simulink model "CF010A_GmTqArbn"  (R2013b)
settings: Solver=FixedStepDiscrete  SolverMode=SingleTasking  StartTime=0.0  StopTime=1  FixedStep=0.002  RelTol=1e-3
values from neighbouring files (symbols this model uses):
  ARCHGLBPRM_2MILLISEC_SEC_F32 = DataDict.Constant    [CF010A_GmTqArbn_DataDict.m]
  ESCTQCMDOVRLLIM_HWNWTMTR_F32 = DataDict.Constant    [CF010A_GmTqArbn_DataDict.m]
  FINALSLEWLWRLIM_HWNWTMTRPERSEC_F32 = DataDict.Constant    [CF010A_GmTqArbn_DataDict.m]
  GmTqArbnApaAssiScaEna = DataDict.Calibration    [CF010A_GmTqArbn_DataDict.m]
  GmTqArbnApaDampgScaEna = DataDict.Calibration    [CF010A_GmTqArbn_DataDict.m]
  GmTqArbnApaEnaRate = DataDict.Calibration    [CF010A_GmTqArbn_DataDict.m]
  GmTqArbnApaRtnScaEna = DataDict.Calibration    [CF010A_GmTqArbn_DataDict.m]
  GmTqArbnEscMaxTq = DataDict.Calibration    [CF010A_GmTqArbn_DataDict.m]
  GmTqArbnLkaOutpOvrlUpprLim = DataDict.Calibration    [CF010A_GmTqArbn_DataDict.m]
  GmTqArbnLkaSlewEna = DataDict.Calibration    [CF010A_GmTqArbn_DataDict.m]
  HWTQCMDOVRLLIM_HWNWTMTR_F32 = DataDict.Constant    [CF010A_GmTqArbn_DataDict.m]
  LKACMDHILIM_HWNWTMTR_F32 = DataDict.Constant    [CF010A_GmTqArbn_DataDict.m]
  LKAOUTPOVRLLIM_MOTNWTMTR_F32 = DataDict.Constant    [CF010A_GmTqArbn_DataDict.m]
  LKATQCMDOVRLLIM_HWNWTMTR_F32 = DataDict.Constant    [CF010A_GmTqArbn_DataDict.m]
  MOTTQCMDOVRLLIM_MOTNWTMTR_F32 = DataDict.Constant    [CF010A_GmTqArbn_DataDict.m]
  OUTPCMDHILIM_ULS_F32 = DataDict.Constant    [CF010A_GmTqArbn_DataDict.m]
  OUTPCMDLOWRLIM_ULS_F32 = DataDict.Constant    [CF010A_GmTqArbn_DataDict.m]
  POSNSERVOSMOOTHMINLWRLIM_ULSPERSEC_F32 = DataDict.Constant    [CF010A_GmTqArbn_DataDict.m]
  VELDPTTQOVRLMTRCOFFS_HWNWTMTRPERSEC_F32 = DataDict.Constant    [CF010A_GmTqArbn_DataDict.m]
  VELDPTTQOVRLMTRCTQPERVEHSPD_HWNWTMTRPERSECPERKPH_F32 = DataDict.Constant    [CF010A_GmTqArbn_DataDict.m]
undefined symbols (not defined in the file or in its folder): GmTqArbnEscSt1, GmTqArbnLkaSt1
libraries: NxtrLim x12, simulink x10, NexteerUtilities x8, FixdToFloat x4, NxtrAbslt x3, Fil x2, FloatToFixd x2, BilnrIntrpnMplX x1, NxtrSign x1
(part 3 of 5)

== system CF010A_GmTqArbn/call_GmTqArbnInit1/Subsystem5 ==

== system CF010A_GmTqArbn/call_GmTqArbnPer1/Subsystem5 ==

== system CF010A_GmTqArbn/GmTqArbn/GmTqArbnInit1/CopyRight2 ==

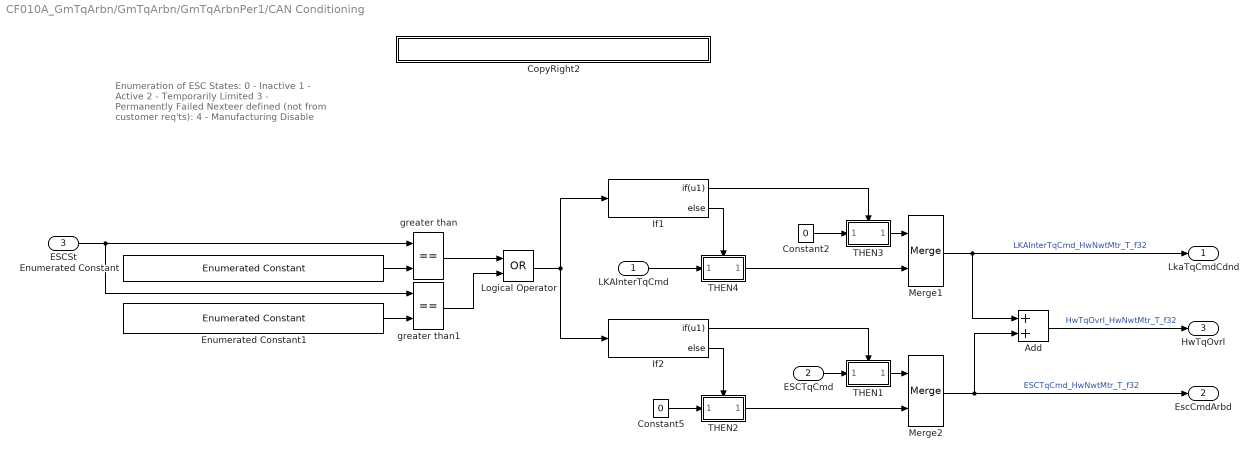
== system CF010A_GmTqArbn/GmTqArbn/GmTqArbnPer1/CAN Conditioning ==
  note: Enumeration of ESC States:
      |     0 - Inactive
      |     1 - Active
      |     2 - Temporarily Limited
      |     3 - Permanently Failed
      |
      | Nexteer defined (not from customer req'ts):
      |     4 - Manufacturing Disable
  LKAInterTqCmd : Inport
  ESCTqCmd : Inport  Port=2
  ESCSt : Inport  Port=3
  Add : Sum
  Constant2 : Constant  Value=0  OutDataTypeStr=single
  Constant5 : Constant  Value=0  OutDataTypeStr=single
  CopyRight2 : Subsystem  Description=|  mask(Copyright Information){none=on}
      | Copyright info block.                                               
      |                                                                     
      | Place copyright information at the top of every subsystem in design.
      mask prompts: none "No parameters"
      mask help: Place copyright information at the top of every subsystem in design.
      mask Display:
      | NxtrConf = 'Nexteer Confidential';
      | 
      | sys = bdroot; %handle for the current model ("system")
      | first = get_param(sys,'Created');
      | first = first(end-3:end);  %year is last four digits
      | 
      | last = get_param(sys,'LastModifiedDate');
      | if isempty(last)
      |     last = datestr(now,'yyyy');
      | else
      |     last = last(end-3:end);
      | end
      | 
      | if strcmp(first,last)
      |     fprintf('%s -- Copyright %s Nexteer',NxtrConf,first)
      | else
      |     fprintf('%s -- %s%s- %s Nexteer',NxtrConf,char(169),first,last)
      | end
  Enumerated Constant : simulink/Sources/Enumerated Constant  OutDataTypeStr=Enum: GmTqArbnEscSt1  Value=GmTqArbnEscSt1.GMTQARBNESCST_ACTV  SampleTime=inf
  Enumerated Constant1 : simulink/Sources/Enumerated Constant  OutDataTypeStr=Enum: GmTqArbnEscSt1  Value=GmTqArbnEscSt1.GMTQARBNESCST_TMPLIMD  SampleTime=inf
  If1 : If  IfExpression=u1
  If2 : If  IfExpression=u1
  Logical Operator : Logic  Operator=OR  AllPortsSameDT=off  OutDataTypeStr=boolean
  Merge1 : Merge
  Merge2 : Merge
  THEN1 : Subsystem  RequirementInfo={} %GIDa_df789066_5626_4b2f_a61b_8784029d3cc8  TreatAsAtomicUnit=on  mask(pass thru, version Nov 30, 2012){nIn=1}
      mask prompts: nIn "Number of input signals"
      mask help:
      | This block passes its input straight through without modification.
      |
      | Enter the number of signals to pass through (integer 1 to 5).
      mask Callback nIn:
      | thisBlock = gcb;
      | a = get_param(thisBlock,'MaskValues');
      | b = cell2mat(a);
      | c = str2num(b);
      | 
      | if c<1 c=1; end
      | if c>5 c=5; end
      | 
      | for idx=1:c
      |     sIdx = num2str(idx);
      |     oldblock = [thisBlock '/In' sIdx];
      |     if strcmp(get_param(oldblock,'BlockType'),'Ground')
      |          newblock = 'built-in/Inport';
      |         pos = get_param(oldblock,'Position');
      |         orient = get_param(oldblock,'Orientation');
      |         delete_block(oldblock);
      |         add_block(newblock,oldblock,'Position',pos, 'Orientation',orient);
      |     end
      | 
      |     oldblock = [thisBlock '/Out' sIdx];
      |     if strcmp(get_param(oldblock,'BlockType'),'Terminator')
      |         newblock = 'built-in/Outport';
      |         pos = get_param(oldblock,'Position');
      |         orient = get_param(oldblock,'Orientation');
      |         delete_block(oldblock);
      |         add_block(newblock,oldblock,'Position',pos, 'Orientation',orient);
      |     end
      | end
      | 
      | for idx=c+1:5
      |     sIdx = num2str(idx);
      |     oldblock = [thisBlock '/In' sIdx];
      |     if strcmp(get_param(oldblock,'BlockType'),'Inport')
      |         newblock = 'built-in/Ground';
      |         pos = get_param(oldblock,'Position');
      |         orient = get_param(oldblock,'Orientation');
      |         delete_block(oldblock);
      |         add_block(newblock,oldblock,'Position',pos, 'Orientation',orient);
      |     end
      | 
      |     oldblock = [thisBlock '/Out' sIdx];
      |     if strcmp(get_param(oldblock,'BlockType'),'Outport')
      |         newblock = 'built-in/Terminator';
      |         pos = get_param(oldblock,'Position');
      |         orient = get_param(oldblock,'Orientation');
      |         delete_block(oldblock);
      |         add_block(newblock,oldblock,'Position',pos, 'Orientation',orient);
      |     end
      | end
      | 
      | 
      | 
      | clear thisBlock oldblock newblock orient pos a b c idx sIdx ;
      mask Display: fprintf('pass\nthru')
  THEN2 : Subsystem  RequirementInfo={} %GIDa_50ca75fe_c393_440b_9fca_2138a66effba  TreatAsAtomicUnit=on  mask(pass thru, version Nov 30, 2012){nIn=1}
      mask prompts: nIn "Number of input signals"
      mask help:
      | This block passes its input straight through without modification.
      |
      | Enter the number of signals to pass through (integer 1 to 5).
      mask Callback nIn:
      | thisBlock = gcb;
      | a = get_param(thisBlock,'MaskValues');
      | b = cell2mat(a);
      | c = str2num(b);
      | 
      | if c<1 c=1; end
      | if c>5 c=5; end
      | 
      | for idx=1:c
      |     sIdx = num2str(idx);
      |     oldblock = [thisBlock '/In' sIdx];
      |     if strcmp(get_param(oldblock,'BlockType'),'Ground')
      |          newblock = 'built-in/Inport';
      |         pos = get_param(oldblock,'Position');
      |         orient = get_param(oldblock,'Orientation');
      |         delete_block(oldblock);
      |         add_block(newblock,oldblock,'Position',pos, 'Orientation',orient);
      |     end
      | 
      |     oldblock = [thisBlock '/Out' sIdx];
      |     if strcmp(get_param(oldblock,'BlockType'),'Terminator')
      |         newblock = 'built-in/Outport';
      |         pos = get_param(oldblock,'Position');
      |         orient = get_param(oldblock,'Orientation');
      |         delete_block(oldblock);
      |         add_block(newblock,oldblock,'Position',pos, 'Orientation',orient);
      |     end
      | end
      | 
      | for idx=c+1:5
      |     sIdx = num2str(idx);
      |     oldblock = [thisBlock '/In' sIdx];
      |     if strcmp(get_param(oldblock,'BlockType'),'Inport')
      |         newblock = 'built-in/Ground';
      |         pos = get_param(oldblock,'Position');
      |         orient = get_param(oldblock,'Orientation');
      |         delete_block(oldblock);
      |         add_block(newblock,oldblock,'Position',pos, 'Orientation',orient);
      |     end
      | 
      |     oldblock = [thisBlock '/Out' sIdx];
      |     if strcmp(get_param(oldblock,'BlockType'),'Outport')
      |         newblock = 'built-in/Terminator';
      |         pos = get_param(oldblock,'Position');
      |         orient = get_param(oldblock,'Orientation');
      |         delete_block(oldblock);
      |         add_block(newblock,oldblock,'Position',pos, 'Orientation',orient);
      |     end
      | end
      | 
      | 
      | 
      | clear thisBlock oldblock newblock orient pos a b c idx sIdx ;
      mask Display: fprintf('pass\nthru')
  THEN3 : Subsystem  RequirementInfo={} %GIDa_81dcbbe4_bcf9_4683_b7ed_1b758c0b3447  TreatAsAtomicUnit=on  mask(pass thru, version Nov 30, 2012){nIn=1}
      mask prompts: nIn "Number of input signals"
      mask help:
      | This block passes its input straight through without modification.
      |
      | Enter the number of signals to pass through (integer 1 to 5).
      mask Callback nIn:
      | thisBlock = gcb;
      | a = get_param(thisBlock,'MaskValues');
      | b = cell2mat(a);
      | c = str2num(b);
      | 
      | if c<1 c=1; end
      | if c>5 c=5; end
      | 
      | for idx=1:c
      |     sIdx = num2str(idx);
      |     oldblock = [thisBlock '/In' sIdx];
      |     if strcmp(get_param(oldblock,'BlockType'),'Ground')
      |          newblock = 'built-in/Inport';
      |         pos = get_param(oldblock,'Position');
      |         orient = get_param(oldblock,'Orientation');
      |         delete_block(oldblock);
      |         add_block(newblock,oldblock,'Position',pos, 'Orientation',orient);
      |     end
      | 
      |     oldblock = [thisBlock '/Out' sIdx];
      |     if strcmp(get_param(oldblock,'BlockType'),'Terminator')
      |         newblock = 'built-in/Outport';
      |         pos = get_param(oldblock,'Position');
      |         orient = get_param(oldblock,'Orientation');
      |         delete_block(oldblock);
      |         add_block(newblock,oldblock,'Position',pos, 'Orientation',orient);
      |     end
      | end
      | 
      | for idx=c+1:5
      |     sIdx = num2str(idx);
      |     oldblock = [thisBlock '/In' sIdx];
      |     if strcmp(get_param(oldblock,'BlockType'),'Inport')
      |         newblock = 'built-in/Ground';
      |         pos = get_param(oldblock,'Position');
      |         orient = get_param(oldblock,'Orientation');
      |         delete_block(oldblock);
      |         add_block(newblock,oldblock,'Position',pos, 'Orientation',orient);
      |     end
      | 
      |     oldblock = [thisBlock '/Out' sIdx];
      |     if strcmp(get_param(oldblock,'BlockType'),'Outport')
      |         newblock = 'built-in/Terminator';
      |         pos = get_param(oldblock,'Position');
      |         orient = get_param(oldblock,'Orientation');
      |         delete_block(oldblock);
      |         add_block(newblock,oldblock,'Position',pos, 'Orientation',orient);
      |     end
      | end
      | 
      | 
      | 
      | clear thisBlock oldblock newblock orient pos a b c idx sIdx ;
      mask Display: fprintf('pass\nthru')
  THEN4 : Subsystem  RequirementInfo={} %GIDa_7b8aef20_5d37_42b0_b34b_35905273f895  TreatAsAtomicUnit=on  mask(pass thru, version Nov 30, 2012){nIn=1}
      mask prompts: nIn "Number of input signals"
      mask help:
      | This block passes its input straight through without modification.
      |
      | Enter the number of signals to pass through (integer 1 to 5).
      mask Callback nIn:
      | thisBlock = gcb;
      | a = get_param(thisBlock,'MaskValues');
      | b = cell2mat(a);
      | c = str2num(b);
      | 
      | if c<1 c=1; end
      | if c>5 c=5; end
      | 
      | for idx=1:c
      |     sIdx = num2str(idx);
      |     oldblock = [thisBlock '/In' sIdx];
      |     if strcmp(get_param(oldblock,'BlockType'),'Ground')
      |          newblock = 'built-in/Inport';
      |         pos = get_param(oldblock,'Position');
      |         orient = get_param(oldblock,'Orientation');
      |         delete_block(oldblock);
      |         add_block(newblock,oldblock,'Position',pos, 'Orientation',orient);
      |     end
      | 
      |     oldblock = [thisBlock '/Out' sIdx];
      |     if strcmp(get_param(oldblock,'BlockType'),'Terminator')
      |         newblock = 'built-in/Outport';
      |         pos = get_param(oldblock,'Position');
      |         orient = get_param(oldblock,'Orientation');
      |         delete_block(oldblock);
      |         add_block(newblock,oldblock,'Position',pos, 'Orientation',orient);
      |     end
      | end
      | 
      | for idx=c+1:5
      |     sIdx = num2str(idx);
      |     oldblock = [thisBlock '/In' sIdx];
      |     if strcmp(get_param(oldblock,'BlockType'),'Inport')
      |         newblock = 'built-in/Ground';
      |         pos = get_param(oldblock,'Position');
      |         orient = get_param(oldblock,'Orientation');
      |         delete_block(oldblock);
      |         add_block(newblock,oldblock,'Position',pos, 'Orientation',orient);
      |     end
      | 
      |     oldblock = [thisBlock '/Out' sIdx];
      |     if strcmp(get_param(oldblock,'BlockType'),'Outport')
      |         newblock = 'built-in/Terminator';
      |         pos = get_param(oldblock,'Position');
      |         orient = get_param(oldblock,'Orientation');
      |         delete_block(oldblock);
      |         add_block(newblock,oldblock,'Position',pos, 'Orientation',orient);
      |     end
      | end
      | 
      | 
      | 
      | clear thisBlock oldblock newblock orient pos a b c idx sIdx ;
      mask Display: fprintf('pass\nthru')
  greater than : RelationalOperator  Operator===  OutDataTypeStr=boolean
  greater than1 : RelationalOperator  Operator===  OutDataTypeStr=boolean
  LkaTqCmdCdnd : Outport
  EscCmdArbd : Outport  Port=2
  HwTqOvrl : Outport  Port=3
  wires:
  ESCSt/1 -> greater than1/1, greater than/1
  greater than/1 -> Logical Operator/1
  greater than1/1 -> Logical Operator/2
  THEN3/1(Out1) -> Merge1/1
  Constant2/1 -> THEN3/1(In1)
  If1/1 -> THEN3/Action
  LKAInterTqCmd/1 -> THEN4/1(In1)
  If1/2 -> THEN4/Action
  THEN4/1(Out1) -> Merge1/2
  Enumerated Constant/1 -> greater than/2
  Enumerated Constant1/1 -> greater than1/2
  Logical Operator/1 -> If2/1, If1/1
  THEN1/1(Out1) -> Merge2/1
  If2/1 -> THEN1/Action
  If2/2 -> THEN2/Action
  THEN2/1(Out1) -> Merge2/2
  Merge2/1 -> Add/2, EscCmdArbd/1  "ESCTqCmd_HwNwtMtr_T_f32"
  Merge1/1 -> Add/1, LkaTqCmdCdnd/1  "LKAInterTqCmd_HwNwtMtr_T_f32"
  Add/1 -> HwTqOvrl/1  "HwTqOvrl_HwNwtMtr_T_f32"
  ESCTqCmd/1 -> THEN1/1(In1)
  Constant5/1 -> THEN2/1(In1)

== system CF010A_GmTqArbn/GmTqArbn/GmTqArbnPer1/CopyRight2 ==

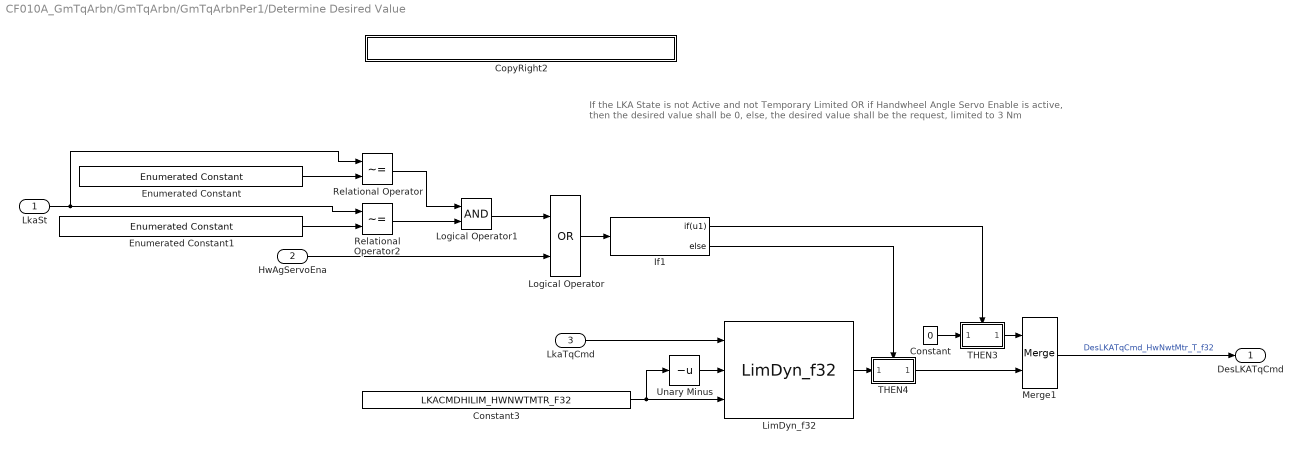
== system CF010A_GmTqArbn/GmTqArbn/GmTqArbnPer1/Determine Desired Value ==
  note: If the LKA State is not Active and not Temporary Limited OR if Handwheel Angle Servo Enable is active, then the desired value shall be 0,
      | else, the desired value shall be the request, limited to 3 Nm
  LkaSt : Inport  RequirementInfo="{'linktype_rmi_doors' '0000c6e3 (/E-STEER Core/SubSystem Specifications/Customer Functions - EA4/GM/CF010A GM Torque Arbitrator)' '#CF010A_80' 'true' 'REQ:  CF010A_80' '' } %GIDa_e9626d04_ec45_4384_8ab6_ba8efd32f7c2"
  HwAgServoEna : Inport  RequirementInfo="{'linktype_rmi_doors' '0000c6e3 (/E-STEER Core/SubSystem Specifications/Customer Functions - EA4/GM/CF010A GM Torque Arbitrator)' '#CF010A_80' 'true' 'REQ:  CF010A_80' '' } %GIDa_c81c3dea_3d6e_4358_9f59_c75afd086a06"  Port=2
  LkaTqCmd : Inport  RequirementInfo="{'linktype_rmi_doors' '0000c6e3 (/E-STEER Core/SubSystem Specifications/Customer Functions - EA4/GM/CF010A GM Torque Arbitrator)' '#CF010A_74' 'true' 'REQ:  CF010A_74' '' } %GIDa_2c9b7aa2_ff43_4516_b45c_8b8c0e299a74"  Port=3
  Constant : Constant  RequirementInfo="{'linktype_rmi_doors' '0000c6e3 (/E-STEER Core/SubSystem Specifications/Customer Functions - EA4/GM/CF010A GM Torque Arbitrator)' '#CF010A_80' 'true' 'REQ:  CF010A_80' '' } %GIDa_2a982d6b_11a7_487a_8418_a7b27190e0d7"  Value=0  OutDataTypeStr=single
  Constant3 : Constant  RequirementInfo="{'linktype_rmi_doors' '0000c6e3 (/E-STEER Core/SubSystem Specifications/Customer Functions - EA4/GM/CF010A GM Torque Arbitrator)' '#CF010A_74' 'true' 'REQ:  CF010A_74' '' } %GIDa_654ca391_7ecf_4f1e_8db5_101135cd2d63"  Value=LKACMDHILIM_HWNWTMTR_F32
  CopyRight2 : Subsystem  Description=|  mask(Copyright Information){none=on}
      | Copyright info block.                                               
      |                                                                     
      | Place copyright information at the top of every subsystem in design.
      mask prompts: none "No parameters"
      mask help: Place copyright information at the top of every subsystem in design.
      mask Display:
      | NxtrConf = 'Nexteer Confidential';
      | 
      | sys = bdroot; %handle for the current model ("system")
      | first = get_param(sys,'Created');
      | first = first(end-3:end);  %year is last four digits
      | 
      | last = get_param(sys,'LastModifiedDate');
      | if isempty(last)
      |     last = datestr(now,'yyyy');
      | else
      |     last = last(end-3:end);
      | end
      | 
      | if strcmp(first,last)
      |     fprintf('%s -- Copyright %s Nexteer',NxtrConf,first)
      | else
      |     fprintf('%s -- %s%s- %s Nexteer',NxtrConf,char(169),first,last)
      | end
  Enumerated Constant : simulink/Sources/Enumerated Constant  RequirementInfo="{'linktype_rmi_doors' '0000c6e3 (/E-STEER Core/SubSystem Specifications/Customer Functions - EA4/GM/CF010A GM Torque Arbitrator)' '#CF010A_80' 'true' 'REQ:  CF010A_80' '' } %GIDa_8e7bdd67_d95a_478f_927e_4ce6c70fd8ed"  OutDataTypeStr=Enum: GmTqArbnLkaSt1  Value=GmTqArbnLkaSt1.GMTQARBNLKAST_ACTV  SampleTime=inf
  Enumerated Constant1 : simulink/Sources/Enumerated Constant  RequirementInfo="{'linktype_rmi_doors' '0000c6e3 (/E-STEER Core/SubSystem Specifications/Customer Functions - EA4/GM/CF010A GM Torque Arbitrator)' '#CF010A_80' 'true' 'REQ:  CF010A_80' '' } %GIDa_f24a38a1_84f5_4752_8e9d_0378cdf66918"  OutDataTypeStr=Enum: GmTqArbnLkaSt1  Value=GmTqArbnLkaSt1.GMTQARBNLKAST_TMPLIMD  SampleTime=inf
  If1 : If  RequirementInfo="{'linktype_rmi_doors' '0000c6e3 (/E-STEER Core/SubSystem Specifications/Customer Functions - EA4/GM/CF010A GM Torque Arbitrator)' '#CF010A_80' 'true' 'REQ:  CF010A_80' '' } %GIDa_8edfc850_3a79_4a71_8b48_352dacd667c7"  IfExpression=u1
  LimDyn_f32 : NxtrLim/LimDyn_f32  RequirementInfo="{'linktype_rmi_doors' '0000c6e3 (/E-STEER Core/SubSystem Specifications/Customer Functions - EA4/GM/CF010A GM Torque Arbitrator)' '#CF010A_74' 'true' 'REQ:  CF010A_74' '' } %GIDa_6296e332_ce84_4f8f_a08b_7a5917ee8b2e"
  Logical Operator : Logic  RequirementInfo="{'linktype_rmi_doors' '0000c6e3 (/E-STEER Core/SubSystem Specifications/Customer Functions - EA4/GM/CF010A GM Torque Arbitrator)' '#CF010A_80' 'true' 'REQ:  CF010A_80' '' } %GIDa_e68e713c_be4f_470f_8515_f592628c8414"  Operator=OR  AllPortsSameDT=off  OutDataTypeStr=boolean
  Logical Operator1 : Logic  AllPortsSameDT=off  OutDataTypeStr=boolean
  Merge1 : Merge  RequirementInfo="{'linktype_rmi_doors' '0000c6e3 (/E-STEER Core/SubSystem Specifications/Customer Functions - EA4/GM/CF010A GM Torque Arbitrator)' '#CF010A_80' 'true' 'REQ:  CF010A_80' '' } %GIDa_7ceb91cf_392d_41c7_b296_9e22297022fe"
  Relational Operator : RelationalOperator  RequirementInfo="{'linktype_rmi_doors' '0000c6e3 (/E-STEER Core/SubSystem Specifications/Customer Functions - EA4/GM/CF010A GM Torque Arbitrator)' '#CF010A_80' 'true' 'REQ:  CF010A_80' '' } %GIDa_1bae5a02_9439_477b_80cb_677fe5a7c8c6"  Operator=~=  OutDataTypeStr=boolean
  Relational Operator2 : RelationalOperator  RequirementInfo="{'linktype_rmi_doors' '0000c6e3 (/E-STEER Core/SubSystem Specifications/Customer Functions - EA4/GM/CF010A GM Torque Arbitrator)' '#CF010A_80' 'true' 'REQ:  CF010A_80' '' } %GIDa_e0135f40_02d3_415f_bca5_0728cc42a656"  Operator=~=  OutDataTypeStr=boolean
  THEN3 : Subsystem  RequirementInfo="{'linktype_rmi_doors' '0000c6e3 (/E-STEER Core/SubSystem Specifications/Customer Functions - EA4/GM/CF010A GM Torque Arbitrator)' '#CF010A_80' 'true' 'REQ:  CF010A_80' '' } %GIDa_0606f6db_8c1b_4172_ad9d_e86aee79a80c"  TreatAsAtomicUnit=on  mask(pass thru, version Nov 30, 2012){nIn=1}
      mask prompts: nIn "Number of input signals"
      mask help:
      | This block passes its input straight through without modification.
      |
      | Enter the number of signals to pass through (integer 1 to 5).
      mask Callback nIn:
      | thisBlock = gcb;
      | a = get_param(thisBlock,'MaskValues');
      | b = cell2mat(a);
      | c = str2num(b);
      | 
      | if c<1 c=1; end
      | if c>5 c=5; end
      | 
      | for idx=1:c
      |     sIdx = num2str(idx);
      |     oldblock = [thisBlock '/In' sIdx];
      |     if strcmp(get_param(oldblock,'BlockType'),'Ground')
      |          newblock = 'built-in/Inport';
      |         pos = get_param(oldblock,'Position');
      |         orient = get_param(oldblock,'Orientation');
      |         delete_block(oldblock);
      |         add_block(newblock,oldblock,'Position',pos, 'Orientation',orient);
      |     end
      | 
      |     oldblock = [thisBlock '/Out' sIdx];
      |     if strcmp(get_param(oldblock,'BlockType'),'Terminator')
      |         newblock = 'built-in/Outport';
      |         pos = get_param(oldblock,'Position');
      |         orient = get_param(oldblock,'Orientation');
      |         delete_block(oldblock);
      |         add_block(newblock,oldblock,'Position',pos, 'Orientation',orient);
      |     end
      | end
      | 
      | for idx=c+1:5
      |     sIdx = num2str(idx);
      |     oldblock = [thisBlock '/In' sIdx];
      |     if strcmp(get_param(oldblock,'BlockType'),'Inport')
      |         newblock = 'built-in/Ground';
      |         pos = get_param(oldblock,'Position');
      |         orient = get_param(oldblock,'Orientation');
      |         delete_block(oldblock);
      |         add_block(newblock,oldblock,'Position',pos, 'Orientation',orient);
      |     end
      | 
      |     oldblock = [thisBlock '/Out' sIdx];
      |     if strcmp(get_param(oldblock,'BlockType'),'Outport')
      |         newblock = 'built-in/Terminator';
      |         pos = get_param(oldblock,'Position');
      |         orient = get_param(oldblock,'Orientation');
      |         delete_block(oldblock);
      |         add_block(newblock,oldblock,'Position',pos, 'Orientation',orient);
      |     end
      | end
      | 
      | 
      | 
      | clear thisBlock oldblock newblock orient pos a b c idx sIdx ;
      mask Display: fprintf('pass\nthru')
  THEN4 : Subsystem  RequirementInfo="{'linktype_rmi_doors' '0000c6e3 (/E-STEER Core/SubSystem Specifications/Customer Functions - EA4/GM/CF010A GM Torque Arbitrator)' '#CF010A_80' 'true' 'REQ:  CF010A_80' '' } %GIDa_83d48c39_410e_4c17_a4dc_2ab1cb247f6f"  TreatAsAtomicUnit=on  mask(pass thru, version Nov 30, 2012){nIn=1}
      mask prompts: nIn "Number of input signals"
      mask help:
      | This block passes its input straight through without modification.
      |
      | Enter the number of signals to pass through (integer 1 to 5).
      mask Callback nIn:
      | thisBlock = gcb;
      | a = get_param(thisBlock,'MaskValues');
      | b = cell2mat(a);
      | c = str2num(b);
      | 
      | if c<1 c=1; end
      | if c>5 c=5; end
      | 
      | for idx=1:c
      |     sIdx = num2str(idx);
      |     oldblock = [thisBlock '/In' sIdx];
      |     if strcmp(get_param(oldblock,'BlockType'),'Ground')
      |          newblock = 'built-in/Inport';
      |         pos = get_param(oldblock,'Position');
      |         orient = get_param(oldblock,'Orientation');
      |         delete_block(oldblock);
      |         add_block(newblock,oldblock,'Position',pos, 'Orientation',orient);
      |     end
      | 
      |     oldblock = [thisBlock '/Out' sIdx];
      |     if strcmp(get_param(oldblock,'BlockType'),'Terminator')
      |         newblock = 'built-in/Outport';
      |         pos = get_param(oldblock,'Position');
      |         orient = get_param(oldblock,'Orientation');
      |         delete_block(oldblock);
      |         add_block(newblock,oldblock,'Position',pos, 'Orientation',orient);
      |     end
      | end
      | 
      | for idx=c+1:5
      |     sIdx = num2str(idx);
      |     oldblock = [thisBlock '/In' sIdx];
      |     if strcmp(get_param(oldblock,'BlockType'),'Inport')
      |         newblock = 'built-in/Ground';
      |         pos = get_param(oldblock,'Position');
      |         orient = get_param(oldblock,'Orientation');
      |         delete_block(oldblock);
      |         add_block(newblock,oldblock,'Position',pos, 'Orientation',orient);
      |     end
      | 
      |     oldblock = [thisBlock '/Out' sIdx];
      |     if strcmp(get_param(oldblock,'BlockType'),'Outport')
      |         newblock = 'built-in/Terminator';
      |         pos = get_param(oldblock,'Position');
      |         orient = get_param(oldblock,'Orientation');
      |         delete_block(oldblock);
      |         add_block(newblock,oldblock,'Position',pos, 'Orientation',orient);
      |     end
      | end
      | 
      | 
      | 
      | clear thisBlock oldblock newblock orient pos a b c idx sIdx ;
      mask Display: fprintf('pass\nthru')
  Unary Minus : UnaryMinus  RequirementInfo="{'linktype_rmi_doors' '0000c6e3 (/E-STEER Core/SubSystem Specifications/Customer Functions - EA4/GM/CF010A GM Torque Arbitrator)' '#CF010A_74' 'true' 'REQ:  CF010A_74' '' } %GIDa_53c20fe0_4aa6_44f8_8aef_48271ea16529"
  DesLKATqCmd : Outport  RequirementInfo="{'linktype_rmi_doors' '0000c6e3 (/E-STEER Core/SubSystem Specifications/Customer Functions - EA4/GM/CF010A GM Torque Arbitrator)' '#CF010A_80' 'true' 'REQ:  CF010A_80' '' } %GIDa_f09ef29e_b286_4ed5_8898_701dc03fd9d3"
  wires:
  HwAgServoEna/1 -> Logical Operator/2
  Logical Operator/1 -> If1/1
  Merge1/1 -> DesLKATqCmd/1  "DesLKATqCmd_HwNwtMtr_T_f32"
  LkaTqCmd/1 -> LimDyn_f32/1
  THEN3/1(Out1) -> Merge1/1
  Constant/1 -> THEN3/1(In1)
  If1/1 -> THEN3/Action
  LimDyn_f32/1 -> THEN4/1(In1)
  If1/2 -> THEN4/Action
  THEN4/1(Out1) -> Merge1/2
  Constant3/1 -> Unary Minus/1, LimDyn_f32/3
  Unary Minus/1 -> LimDyn_f32/2
  Enumerated Constant/1 -> Relational Operator/2
  Logical Operator1/1 -> Logical Operator/1
  Relational Operator/1 -> Logical Operator1/1
  Enumerated Constant1/1 -> Relational Operator2/2
  Relational Operator2/1 -> Logical Operator1/2
  LkaSt/1 -> Relational Operator/1, Relational Operator2/1

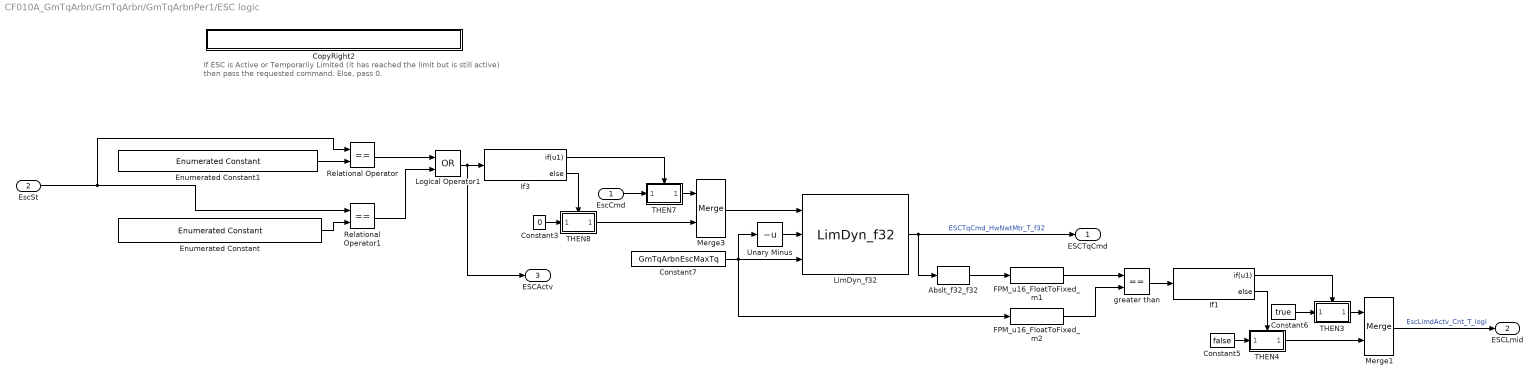
== system CF010A_GmTqArbn/GmTqArbn/GmTqArbnPer1/ESC logic ==
  note: If ESC is Active or Temporarily Limited (it has reached the limit but is still active)
      |   then pass the requested command.
      | Else,
      |   pass 0.
  EscCmd : Inport  RequirementInfo="{'linktype_rmi_doors' '0000c6e3 (/E-STEER Core/SubSystem Specifications/Customer Functions - EA4/GM/CF010A GM Torque Arbitrator)' '#CF010A_77' 'true' 'REQ:  CF010A_77' '' } %GIDa_292744fc_3224_46c7_997d_d7083ceec4be"
  EscSt : Inport  RequirementInfo="{'linktype_rmi_doors' '0000c6e3 (/E-STEER Core/SubSystem Specifications/Customer Functions - EA4/GM/CF010A GM Torque Arbitrator)' '#CF010A_77' 'true' 'REQ:  CF010A_77' '' } %GIDa_6fe11058_23e0_4de6_a7b6_e2eb97c9ca63"  Port=2
  Abslt_f32_f32 : NxtrAbslt/Abslt_f32_f32  RequirementInfo="{'linktype_rmi_doors' '0000c6e3 (/E-STEER Core/SubSystem Specifications/Customer Functions - EA4/GM/CF010A GM Torque Arbitrator)' '#CF010A_82' 'true' 'REQ:  CF010A_82' '' } %GIDa_56a5e4f5_0908_4c61_908f_d3c7880ebc10"  SFunctionSpec=single y1 = Abslt_f32_f32(single u1)
      settings: AttributesFormatString=%<Name>
  Constant3 : Constant  RequirementInfo="{'linktype_rmi_doors' '0000c6e3 (/E-STEER Core/SubSystem Specifications/Customer Functions - EA4/GM/CF010A GM Torque Arbitrator)' '#CF010A_77' 'true' 'REQ:  CF010A_77' '' } %GIDa_e5db8078_2541_46b2_b603_c4888206eaaf"  Value=0  OutDataTypeStr=single
  Constant5 : Constant  RequirementInfo="{'linktype_rmi_doors' '0000c6e3 (/E-STEER Core/SubSystem Specifications/Customer Functions - EA4/GM/CF010A GM Torque Arbitrator)' '#CF010A_82' 'true' 'REQ:  CF010A_82' '' } %GIDa_fa1d5fb8_780a_46bb_aa9a_6854bed56334"  Value=false  OutDataTypeStr=boolean
  Constant6 : Constant  RequirementInfo="{'linktype_rmi_doors' '0000c6e3 (/E-STEER Core/SubSystem Specifications/Customer Functions - EA4/GM/CF010A GM Torque Arbitrator)' '#CF010A_82' 'true' 'REQ:  CF010A_82' '' } %GIDa_d686cdc3_ff37_4ffe_b348_c650d5a0678a"  Value=true  OutDataTypeStr=boolean
  Constant7 : Constant  RequirementInfo="{'linktype_rmi_doors' '0000c6e3 (/E-STEER Core/SubSystem Specifications/Customer Functions - EA4/GM/CF010A GM Torque Arbitrator)' '#CF010A_73' 'true' 'REQ:  CF010A_73' '' } %GIDa_cb46759a_ee61_4af9_8c0b_1010e0cc744b"  Value=GmTqArbnEscMaxTq
  CopyRight2 : Subsystem  Description=|  mask(Copyright Information){none=on}
      | Copyright info block.                                               
      |                                                                     
      | Place copyright information at the top of every subsystem in design.
      mask prompts: none "No parameters"
      mask help: Place copyright information at the top of every subsystem in design.
      mask Display:
      | NxtrConf = 'Nexteer Confidential';
      | 
      | sys = bdroot; %handle for the current model ("system")
      | first = get_param(sys,'Created');
      | first = first(end-3:end);  %year is last four digits
      | 
      | last = get_param(sys,'LastModifiedDate');
      | if isempty(last)
      |     last = datestr(now,'yyyy');
      | else
      |     last = last(end-3:end);
      | end
      | 
      | if strcmp(first,last)
      |     fprintf('%s -- Copyright %s Nexteer',NxtrConf,first)
      | else
      |     fprintf('%s -- %s%s- %s Nexteer',NxtrConf,char(169),first,last)
      | end
  Enumerated Constant : simulink/Sources/Enumerated Constant  RequirementInfo="{'linktype_rmi_doors' '0000c6e3 (/E-STEER Core/SubSystem Specifications/Customer Functions - EA4/GM/CF010A GM Torque Arbitrator)' '#CF010A_77' 'true' 'REQ:  CF010A_77' '' } %GIDa_6527e16e_cd30_442b_a415_e3e0e44159f1"  OutDataTypeStr=Enum: GmTqArbnEscSt1  Value=GmTqArbnEscSt1.GMTQARBNESCST_TMPLIMD  SampleTime=inf
  Enumerated Constant1 : simulink/Sources/Enumerated Constant  RequirementInfo="{'linktype_rmi_doors' '0000c6e3 (/E-STEER Core/SubSystem Specifications/Customer Functions - EA4/GM/CF010A GM Torque Arbitrator)' '#CF010A_77' 'true' 'REQ:  CF010A_77' '' } %GIDa_fd27e72e_74a4_4eee_9057_bd8af7ad7bb5"  OutDataTypeStr=Enum: GmTqArbnEscSt1  Value=GmTqArbnEscSt1.GMTQARBNESCST_ACTV  SampleTime=inf
  FPM_u16_FloatToFixed_m1 : NexteerUtilities/Fixed Point Math Conversions/FPM_u16_FloatToFixed_m  RequirementInfo="{'linktype_rmi_doors' '0000c6e3 (/E-STEER Core/SubSystem Specifications/Customer Functions - EA4/GM/CF010A GM Torque Arbitrator)' '#CF010A_82' 'true' 'REQ:  CF010A_82' '' } %GIDa_9a8f58b3_b098_4328_ad36_d50d0f121c9b"  SFunctionSpec=uint16 y1 = FPM_u16_FloatToFixed_m(single u1, single p1)  Param1=13
      settings: AttributesFormatString=u16_FloatToFixed
  FPM_u16_FloatToFixed_m2 : NexteerUtilities/Fixed Point Math Conversions/FPM_u16_FloatToFixed_m  RequirementInfo="{'linktype_rmi_doors' '0000c6e3 (/E-STEER Core/SubSystem Specifications/Customer Functions - EA4/GM/CF010A GM Torque Arbitrator)' '#CF010A_82' 'true' 'REQ:  CF010A_82' '' } %GIDa_4f626398_9646_414d_86ae_3d26d5603112"  SFunctionSpec=uint16 y1 = FPM_u16_FloatToFixed_m(single u1, single p1)  Param1=13
      settings: AttributesFormatString=u16_FloatToFixed
  If1 : If  RequirementInfo="{'linktype_rmi_doors' '0000c6e3 (/E-STEER Core/SubSystem Specifications/Customer Functions - EA4/GM/CF010A GM Torque Arbitrator)' '#CF010A_82' 'true' 'REQ:  CF010A_82' '' } %GIDa_2c245933_53f1_46e0_bcef_1c4c6fa5e212"  IfExpression=u1
  If3 : If  RequirementInfo="{'linktype_rmi_doors' '0000c6e3 (/E-STEER Core/SubSystem Specifications/Customer Functions - EA4/GM/CF010A GM Torque Arbitrator)' '#CF010A_77' 'true' 'REQ:  CF010A_77' '' } %GIDa_862f68b1_7b77_44bf_bf79_2f384bd96f0f"  IfExpression=u1
  LimDyn_f32 : NxtrLim/LimDyn_f32  RequirementInfo="{'linktype_rmi_doors' '0000c6e3 (/E-STEER Core/SubSystem Specifications/Customer Functions - EA4/GM/CF010A GM Torque Arbitrator)' '#CF010A_73' 'true' 'REQ:  CF010A_73' '' } %GIDa_446e3c56_43d3_4c1e_a90e_b24b8dc02388"
  Logical Operator1 : Logic  RequirementInfo="{'linktype_rmi_doors' '0000c6e3 (/E-STEER Core/SubSystem Specifications/Customer Functions - EA4/GM/CF010A GM Torque Arbitrator)' '#CF010A_77' 'true' 'REQ:  CF010A_77' '' } %GIDa_7bc7e89e_c4bb_42a7_8346_9225a001f5cf"  Operator=OR  AllPortsSameDT=off  OutDataTypeStr=boolean
  Merge1 : Merge  RequirementInfo="{'linktype_rmi_doors' '0000c6e3 (/E-STEER Core/SubSystem Specifications/Customer Functions - EA4/GM/CF010A GM Torque Arbitrator)' '#CF010A_82' 'true' 'REQ:  CF010A_82' '' } %GIDa_0e425789_338d_49c4_81a3_5d5d0fae8ad2"
  Merge3 : Merge  RequirementInfo="{'linktype_rmi_doors' '0000c6e3 (/E-STEER Core/SubSystem Specifications/Customer Functions - EA4/GM/CF010A GM Torque Arbitrator)' '#CF010A_77' 'true' 'REQ:  CF010A_77' '' } %GIDa_72e88514_efc3_45e9_b1e1_1cf5308d120c"
  Relational Operator : RelationalOperator  RequirementInfo="{'linktype_rmi_doors' '0000c6e3 (/E-STEER Core/SubSystem Specifications/Customer Functions - EA4/GM/CF010A GM Torque Arbitrator)' '#CF010A_77' 'true' 'REQ:  CF010A_77' '' } %GIDa_4a32a64c_74e8_498f_83f7_2b86f1c97ccf"  Operator===  OutDataTypeStr=boolean
  Relational Operator1 : RelationalOperator  RequirementInfo="{'linktype_rmi_doors' '0000c6e3 (/E-STEER Core/SubSystem Specifications/Customer Functions - EA4/GM/CF010A GM Torque Arbitrator)' '#CF010A_77' 'true' 'REQ:  CF010A_77' '' } %GIDa_f47b9c17_a8ed_466d_a6e5_43a08d45fb3d"  Operator===  OutDataTypeStr=boolean
  THEN3 : Subsystem  RequirementInfo="{'linktype_rmi_doors' '0000c6e3 (/E-STEER Core/SubSystem Specifications/Customer Functions - EA4/GM/CF010A GM Torque Arbitrator)' '#CF010A_82' 'true' 'REQ:  CF010A_82' '' } %GIDa_7cb0b7aa_377c_45b6_abd8_3cab6ad4e216"  TreatAsAtomicUnit=on  mask(pass thru, version Nov 30, 2012){nIn=1}
      mask prompts: nIn "Number of input signals"
      mask help:
      | This block passes its input straight through without modification.
      |
      | Enter the number of signals to pass through (integer 1 to 5).
      mask Callback nIn:
      | thisBlock = gcb;
      | a = get_param(thisBlock,'MaskValues');
      | b = cell2mat(a);
      | c = str2num(b);
      | 
      | if c<1 c=1; end
      | if c>5 c=5; end
      | 
      | for idx=1:c
      |     sIdx = num2str(idx);
      |     oldblock = [thisBlock '/In' sIdx];
      |     if strcmp(get_param(oldblock,'BlockType'),'Ground')
      |          newblock = 'built-in/Inport';
      |         pos = get_param(oldblock,'Position');
      |         orient = get_param(oldblock,'Orientation');
      |         delete_block(oldblock);
      |         add_block(newblock,oldblock,'Position',pos, 'Orientation',orient);
      |     end
      | 
      |     oldblock = [thisBlock '/Out' sIdx];
      |     if strcmp(get_param(oldblock,'BlockType'),'Terminator')
      |         newblock = 'built-in/Outport';
      |         pos = get_param(oldblock,'Position');
      |         orient = get_param(oldblock,'Orientation');
      |         delete_block(oldblock);
      |         add_block(newblock,oldblock,'Position',pos, 'Orientation',orient);
      |     end
      | end
      | 
      | for idx=c+1:5
      |     sIdx = num2str(idx);
      |     oldblock = [thisBlock '/In' sIdx];
      |     if strcmp(get_param(oldblock,'BlockType'),'Inport')
      |         newblock = 'built-in/Ground';
      |         pos = get_param(oldblock,'Position');
      |         orient = get_param(oldblock,'Orientation');
      |         delete_block(oldblock);
      |         add_block(newblock,oldblock,'Position',pos, 'Orientation',orient);
      |     end
      | 
      |     oldblock = [thisBlock '/Out' sIdx];
      |     if strcmp(get_param(oldblock,'BlockType'),'Outport')
      |         newblock = 'built-in/Terminator';
      |         pos = get_param(oldblock,'Position');
      |         orient = get_param(oldblock,'Orientation');
      |         delete_block(oldblock);
      |         add_block(newblock,oldblock,'Position',pos, 'Orientation',orient);
      |     end
      | end
      | 
      | 
      | 
      | clear thisBlock oldblock newblock orient pos a b c idx sIdx ;
      mask Display: fprintf('pass\nthru')
  THEN4 : Subsystem  RequirementInfo="{'linktype_rmi_doors' '0000c6e3 (/E-STEER Core/SubSystem Specifications/Customer Functions - EA4/GM/CF010A GM Torque Arbitrator)' '#CF010A_82' 'true' 'REQ:  CF010A_82' '' } %GIDa_ec69e255_cda7_4831_824b_afe7668fc332"  TreatAsAtomicUnit=on  mask(pass thru, version Nov 30, 2012){nIn=1}
      mask prompts: nIn "Number of input signals"
      mask help:
      | This block passes its input straight through without modification.
      |
      | Enter the number of signals to pass through (integer 1 to 5).
      mask Callback nIn:
      | thisBlock = gcb;
      | a = get_param(thisBlock,'MaskValues');
      | b = cell2mat(a);
      | c = str2num(b);
      | 
      | if c<1 c=1; end
      | if c>5 c=5; end
      | 
      | for idx=1:c
      |     sIdx = num2str(idx);
      |     oldblock = [thisBlock '/In' sIdx];
      |     if strcmp(get_param(oldblock,'BlockType'),'Ground')
      |          newblock = 'built-in/Inport';
      |         pos = get_param(oldblock,'Position');
      |         orient = get_param(oldblock,'Orientation');
      |         delete_block(oldblock);
      |         add_block(newblock,oldblock,'Position',pos, 'Orientation',orient);
      |     end
      | 
      |     oldblock = [thisBlock '/Out' sIdx];
      |     if strcmp(get_param(oldblock,'BlockType'),'Terminator')
      |         newblock = 'built-in/Outport';
      |         pos = get_param(oldblock,'Position');
      |         orient = get_param(oldblock,'Orientation');
      |         delete_block(oldblock);
      |         add_block(newblock,oldblock,'Position',pos, 'Orientation',orient);
      |     end
      | end
      | 
      | for idx=c+1:5
      |     sIdx = num2str(idx);
      |     oldblock = [thisBlock '/In' sIdx];
      |     if strcmp(get_param(oldblock,'BlockType'),'Inport')
      |         newblock = 'built-in/Ground';
      |         pos = get_param(oldblock,'Position');
      |         orient = get_param(oldblock,'Orientation');
      |         delete_block(oldblock);
      |         add_block(newblock,oldblock,'Position',pos, 'Orientation',orient);
      |     end
      | 
      |     oldblock = [thisBlock '/Out' sIdx];
      |     if strcmp(get_param(oldblock,'BlockType'),'Outport')
      |         newblock = 'built-in/Terminator';
      |         pos = get_param(oldblock,'Position');
      |         orient = get_param(oldblock,'Orientation');
      |         delete_block(oldblock);
      |         add_block(newblock,oldblock,'Position',pos, 'Orientation',orient);
      |     end
      | end
      | 
      | 
      | 
      | clear thisBlock oldblock newblock orient pos a b c idx sIdx ;
      mask Display: fprintf('pass\nthru')
  THEN7 : Subsystem  RequirementInfo="{'linktype_rmi_doors' '0000c6e3 (/E-STEER Core/SubSystem Specifications/Customer Functions - EA4/GM/CF010A GM Torque Arbitrator)' '#CF010A_77' 'true' 'REQ:  CF010A_77' '' } %GIDa_df5e48f9_4d3d_4963_bded_9993ee7d5991"  TreatAsAtomicUnit=on  mask(pass thru, version Nov 30, 2012){nIn=1}
      mask prompts: nIn "Number of input signals"
      mask help:
      | This block passes its input straight through without modification.
      |
      | Enter the number of signals to pass through (integer 1 to 5).
      mask Callback nIn:
      | thisBlock = gcb;
      | a = get_param(thisBlock,'MaskValues');
      | b = cell2mat(a);
      | c = str2num(b);
      | 
      | if c<1 c=1; end
      | if c>5 c=5; end
      | 
      | for idx=1:c
      |     sIdx = num2str(idx);
      |     oldblock = [thisBlock '/In' sIdx];
      |     if strcmp(get_param(oldblock,'BlockType'),'Ground')
      |          newblock = 'built-in/Inport';
      |         pos = get_param(oldblock,'Position');
      |         orient = get_param(oldblock,'Orientation');
      |         delete_block(oldblock);
      |         add_block(newblock,oldblock,'Position',pos, 'Orientation',orient);
      |     end
      | 
      |     oldblock = [thisBlock '/Out' sIdx];
      |     if strcmp(get_param(oldblock,'BlockType'),'Terminator')
      |         newblock = 'built-in/Outport';
      |         pos = get_param(oldblock,'Position');
      |         orient = get_param(oldblock,'Orientation');
      |         delete_block(oldblock);
      |         add_block(newblock,oldblock,'Position',pos, 'Orientation',orient);
      |     end
      | end
      | 
      | for idx=c+1:5
      |     sIdx = num2str(idx);
      |     oldblock = [thisBlock '/In' sIdx];
      |     if strcmp(get_param(oldblock,'BlockType'),'Inport')
      |         newblock = 'built-in/Ground';
      |         pos = get_param(oldblock,'Position');
      |         orient = get_param(oldblock,'Orientation');
      |         delete_block(oldblock);
      |         add_block(newblock,oldblock,'Position',pos, 'Orientation',orient);
      |     end
      | 
      |     oldblock = [thisBlock '/Out' sIdx];
      |     if strcmp(get_param(oldblock,'BlockType'),'Outport')
      |         newblock = 'built-in/Terminator';
      |         pos = get_param(oldblock,'Position');
      |         orient = get_param(oldblock,'Orientation');
      |         delete_block(oldblock);
      |         add_block(newblock,oldblock,'Position',pos, 'Orientation',orient);
      |     end
      | end
      | 
      | 
      | 
      | clear thisBlock oldblock newblock orient pos a b c idx sIdx ;
      mask Display: fprintf('pass\nthru')
  THEN8 : Subsystem  RequirementInfo="{'linktype_rmi_doors' '0000c6e3 (/E-STEER Core/SubSystem Specifications/Customer Functions - EA4/GM/CF010A GM Torque Arbitrator)' '#CF010A_77' 'true' 'REQ:  CF010A_77' '' } %GIDa_058d061c_9a6a_4e56_a7df_5107ed3b1fbe"  TreatAsAtomicUnit=on  mask(pass thru, version Nov 30, 2012){nIn=1}
      mask prompts: nIn "Number of input signals"
      mask help:
      | This block passes its input straight through without modification.
      |
      | Enter the number of signals to pass through (integer 1 to 5).
      mask Callback nIn:
      | thisBlock = gcb;
      | a = get_param(thisBlock,'MaskValues');
      | b = cell2mat(a);
      | c = str2num(b);
      | 
      | if c<1 c=1; end
      | if c>5 c=5; end
      | 
      | for idx=1:c
      |     sIdx = num2str(idx);
      |     oldblock = [thisBlock '/In' sIdx];
      |     if strcmp(get_param(oldblock,'BlockType'),'Ground')
      |          newblock = 'built-in/Inport';
      |         pos = get_param(oldblock,'Position');
      |         orient = get_param(oldblock,'Orientation');
      |         delete_block(oldblock);
      |         add_block(newblock,oldblock,'Position',pos, 'Orientation',orient);
      |     end
      | 
      |     oldblock = [thisBlock '/Out' sIdx];
      |     if strcmp(get_param(oldblock,'BlockType'),'Terminator')
      |         newblock = 'built-in/Outport';
      |         pos = get_param(oldblock,'Position');
      |         orient = get_param(oldblock,'Orientation');
      |         delete_block(oldblock);
      |         add_block(newblock,oldblock,'Position',pos, 'Orientation',orient);
      |     end
      | end
      | 
      | for idx=c+1:5
      |     sIdx = num2str(idx);
      |     oldblock = [thisBlock '/In' sIdx];
      |     if strcmp(get_param(oldblock,'BlockType'),'Inport')
      |         newblock = 'built-in/Ground';
      |         pos = get_param(oldblock,'Position');
      |         orient = get_param(oldblock,'Orientation');
      |         delete_block(oldblock);
      |         add_block(newblock,oldblock,'Position',pos, 'Orientation',orient);
      |     end
      | 
      |     oldblock = [thisBlock '/Out' sIdx];
      |     if strcmp(get_param(oldblock,'BlockType'),'Outport')
      |         newblock = 'built-in/Terminator';
      |         pos = get_param(oldblock,'Position');
      |         orient = get_param(oldblock,'Orientation');
      |         delete_block(oldblock);
      |         add_block(newblock,oldblock,'Position',pos, 'Orientation',orient);
      |     end
      | end
      | 
      | 
      | 
      | clear thisBlock oldblock newblock orient pos a b c idx sIdx ;
      mask Display: fprintf('pass\nthru')
  Unary Minus : UnaryMinus  RequirementInfo="{'linktype_rmi_doors' '0000c6e3 (/E-STEER Core/SubSystem Specifications/Customer Functions - EA4/GM/CF010A GM Torque Arbitrator)' '#CF010A_73' 'true' 'REQ:  CF010A_73' '' } %GIDa_106b8bb5_ea8f_4824_915d_b6fc8fdda4b4"
  greater than : RelationalOperator  RequirementInfo="{'linktype_rmi_doors' '0000c6e3 (/E-STEER Core/SubSystem Specifications/Customer Functions - EA4/GM/CF010A GM Torque Arbitrator)' '#CF010A_82' 'true' 'REQ:  CF010A_82' '' } %GIDa_bf3560f0_1c15_4279_8fe6_1460799041a4"  Operator===  OutDataTypeStr=boolean
  ESCTqCmd : Outport  RequirementInfo="{'linktype_rmi_doors' '0000c6e3 (/E-STEER Core/SubSystem Specifications/Customer Functions - EA4/GM/CF010A GM Torque Arbitrator)' '#CF010A_77' 'true' 'REQ:  CF010A_77' '' } %GIDa_49f5c37b_dd32_49ef_b2db_bb0486673fcd"
  ESCLmid : Outport  RequirementInfo="{'linktype_rmi_doors' '0000c6e3 (/E-STEER Core/SubSystem Specifications/Customer Functions - EA4/GM/CF010A GM Torque Arbitrator)' '#CF010A_82' 'true' 'REQ:  CF010A_82' '' } %GIDa_dd64d4f7_ef9c_4db6_8ab4_c21110062263"  Port=2
  ESCActv : Outport  RequirementInfo="{'linktype_rmi_doors' '0000c6e3 (/E-STEER Core/SubSystem Specifications/Customer Functions - EA4/GM/CF010A GM Torque Arbitrator)' '#CF010A_113' 'true' 'REQ:  CF010A_113' '' } %GIDa_813dea43_b87c_41f7_b3d2_86e0621b2197"  Port=3
  wires:
  Abslt_f32_f32/1 -> FPM_u16_FloatToFixed_m1/1
  EscSt/1 -> Relational Operator/1, Relational Operator1/1
  Relational Operator/1 -> Logical Operator1/1
  Relational Operator1/1 -> Logical Operator1/2
  Logical Operator1/1 -> ESCActv/1, If3/1
  Merge1/1 -> ESCLmid/1  "EscLimdActv_Cnt_T_logl"
  LimDyn_f32/1 -> Abslt_f32_f32/1, ESCTqCmd/1  "ESCTqCmd_HwNwtMtr_T_f32"
  Enumerated Constant1/1 -> Relational Operator/2
  Enumerated Constant/1 -> Relational Operator1/2
  THEN7/1(Out1) -> Merge3/1
  EscCmd/1 -> THEN7/1(In1)
  If3/1 -> THEN7/Action
  Constant3/1 -> THEN8/1(In1)
  If3/2 -> THEN8/Action
  THEN8/1(Out1) -> Merge3/2
  Constant7/1 -> FPM_u16_FloatToFixed_m2/1, Unary Minus/1, LimDyn_f32/3
  THEN3/1(Out1) -> Merge1/1
  Constant6/1 -> THEN3/1(In1)
  If1/1 -> THEN3/Action
  Constant5/1 -> THEN4/1(In1)
  If1/2 -> THEN4/Action
  THEN4/1(Out1) -> Merge1/2
  greater than/1 -> If1/1
  Merge3/1 -> LimDyn_f32/1
  Unary Minus/1 -> LimDyn_f32/2
  FPM_u16_FloatToFixed_m1/1 -> greater than/1
  FPM_u16_FloatToFixed_m2/1 -> greater than/2
